simulink model "model"  (R2022b)
settings: Solver=VariableStepAuto  StartTime=0.0  StopTime=10.0  RelTol=1e-3
settings Model: Creator=hayden  LastModifiedBy=hayden

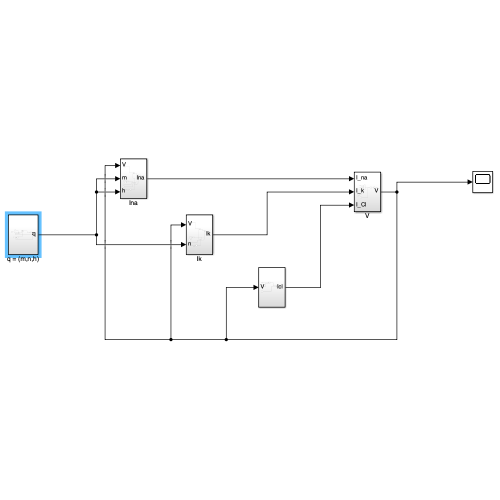
[thumbnail: Simulink's stored preview of the top-level diagram]
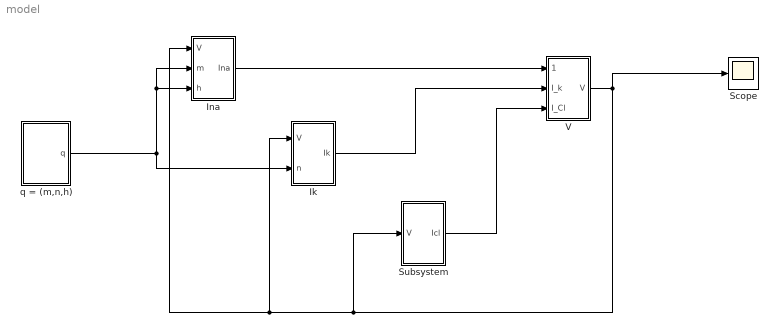
== system model ==
  Ik : Subsystem
  Ina : Subsystem
  Scope : Scope
  Subsystem : Subsystem
  V : Subsystem
  q = (m,n,h) : Subsystem
  wires:
  V/1(V) -> Scope/1, Subsystem/1(V), Ik/1(V), Ina/1(V)
  Subsystem/1(Icl) -> V/3(I_Cl)
  Ik/1(Ik) -> V/2(I_k)
  Ina/1(Ina) -> V/1(I_na)
  q = (m,n,h)/1(q) -> Ik/2(n), Ina/3(h), Ina/2(m)

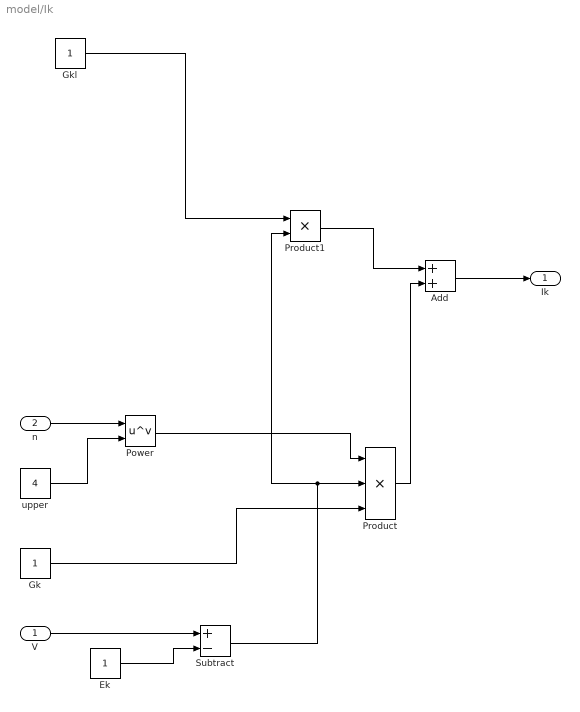
== system model/Ik ==
  V : Inport
  n : Inport  Port=2
  Add : Sum
  Ek : Constant
  Gk : Constant
  Gkl : Constant
  Power : Math  Operator=pow
  Product : Product  Inputs=3
  Product1 : Product
  Subtract : Sum  Inputs=+-
  upper : Constant  Value=4
  Ik : Outport
  wires:
  Gkl/1 -> Product1/1
  n/1 -> Power/1
  upper/1 -> Power/2
  Power/1 -> Product/1
  Gk/1 -> Product/3
  V/1 -> Subtract/1
  Ek/1 -> Subtract/2
  Subtract/1 -> Product/2, Product1/2
  Product1/1 -> Add/1
  Product/1 -> Add/2
  Add/1 -> Ik/1

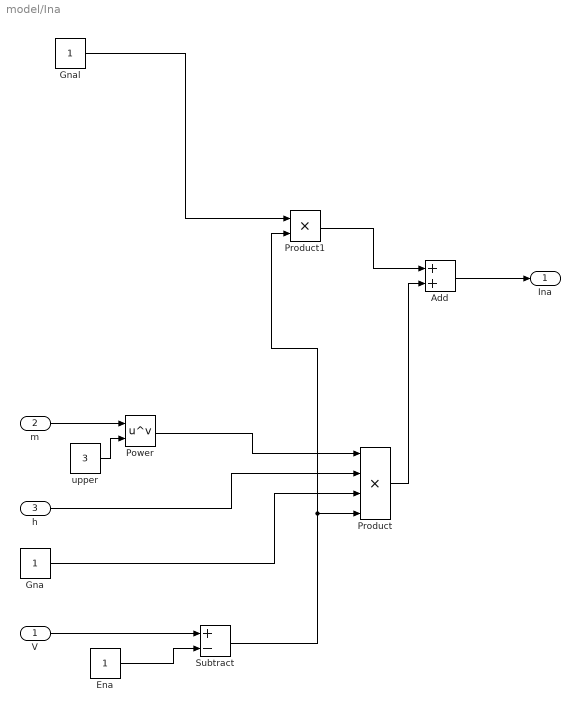
== system model/Ina ==
  V : Inport
  m : Inport  Port=2
  h : Inport  Port=3
  Add : Sum
  Ena : Constant
  Gna : Constant
  Gnal : Constant
  Power : Math  Operator=pow
  Product : Product  Inputs=4
  Product1 : Product
  Subtract : Sum  Inputs=+-
  upper : Constant  Value=3
  Ina : Outport
  wires:
  Gnal/1 -> Product1/1
  m/1 -> Power/1
  upper/1 -> Power/2
  Power/1 -> Product/1
  h/1 -> Product/2
  Gna/1 -> Product/3
  V/1 -> Subtract/1
  Ena/1 -> Subtract/2
  Subtract/1 -> Product1/2, Product/4
  Product1/1 -> Add/1
  Product/1 -> Add/2
  Add/1 -> Ina/1

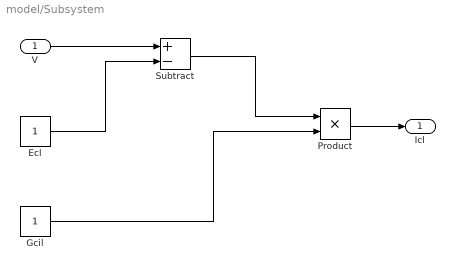
== system model/Subsystem ==
  V : Inport
  Ecl : Constant
  Gcil : Constant
  Product : Product
  Subtract : Sum  Inputs=+-
  Icl : Outport
  wires:
  Product/1 -> Icl/1
  V/1 -> Subtract/1
  Ecl/1 -> Subtract/2
  Gcil/1 -> Product/2
  Subtract/1 -> Product/1

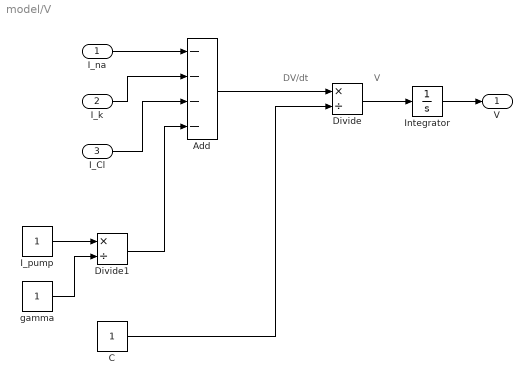
== system model/V ==
  note: V
  note: DV/dt
  I_na : Inport
  I_k : Inport  Port=2
  I_Cl : Inport  Port=3
  Add : Sum  Inputs=----
  C : Constant
  Divide : Product  Inputs=*/
  Divide1 : Product  Inputs=*/
  I_pump : Constant
  Integrator : Integrator
  gamma : Constant
  V : Outport
  wires:
  Integrator/1 -> V/1
  Divide/1 -> Integrator/1
  Add/1 -> Divide/1
  I_na/1 -> Add/1
  I_k/1 -> Add/2
  I_Cl/1 -> Add/3
  C/1 -> Divide/2
  I_pump/1 -> Divide1/1
  gamma/1 -> Divide1/2
  Divide1/1 -> Add/4

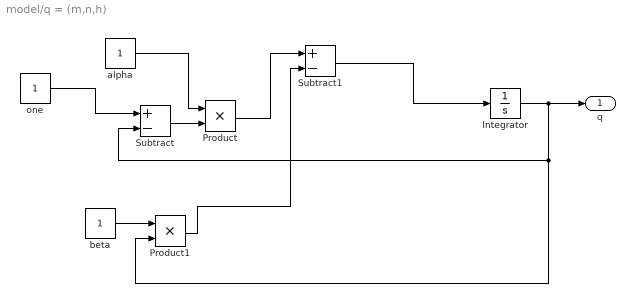
== system model/q = (m,n,h) ==
  Integrator : Integrator
  Product : Product
  Product1 : Product
  Subtract : Sum  Inputs=+-
  Subtract1 : Sum  Inputs=+-
  alpha : Constant
  beta : Constant
  one : Constant
  q : Outport
  wires:
  Integrator/1 -> Product1/2, Subtract/2, q/1
  one/1 -> Subtract/1
  Subtract/1 -> Product/2
  alpha/1 -> Product/1
  Product/1 -> Subtract1/1
  beta/1 -> Product1/1
  Product1/1 -> Subtract1/2
  Subtract1/1 -> Integrator/1
